simulink model "simulare_regulator_etapa2"  (R2020a)
settings: Solver=VariableStepAuto  StartTime=0.0  StopTime=500  RelTol=1e-3
settings Model: Creator=user  LastModifiedBy=user

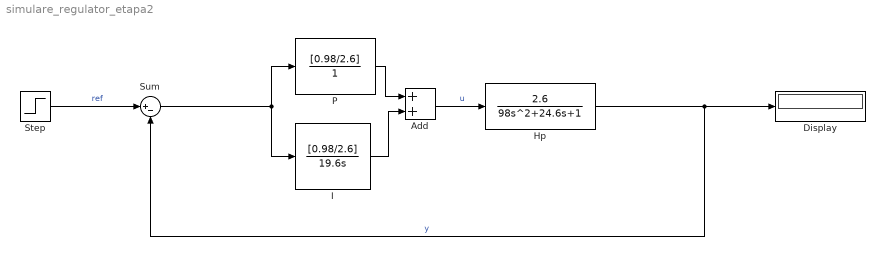
== system simulare_regulator_etapa2 ==
  Add : Sum
  Display : Display
  Hp : TransferFcn  Numerator=[2.6]  Denominator=[98 24.6 1]
  I : TransferFcn  Numerator=[0.98/2.6]  Denominator=[19.6 0]
  P : TransferFcn  Numerator=[0.98/2.6]  Denominator=[0 1]
  Step : Step  SampleTime=0
  Sum : Sum  Inputs=|+-
  wires:
  Step/1 -> Sum/1  "ref"
  Add/1 -> Hp/1  "u"
  Hp/1 -> Sum/2, Display/1  "y"
  P/1 -> Add/1
  I/1 -> Add/2
  Sum/1 -> I/1, P/1
